simulink model "gm_am_demod_hdl_coder"  (R2021b)
settings: Solver=FixedStepAuto  StartTime=0.0  StopTime=20  RelTol=1e-3  EnableMultiTasking=on
libraries: hdlmdlgenlib x10
settings Model: Creator=caccolillo  LastModifiedBy=caccolillo
settings SolverCC: AutoInsertRateTranBlk=on
settings OptimizationCC: BlockReduction=off  ConditionallyExecuteInputs=off  DefaultParameterBehavior=Inlined  UseDivisionForNetSlopeComputation=on  GainParamInheritBuiltInType=on  UseFloatMulNetSlope=on  InlineInvariantSignals=on  EfficientFloat2IntCast=on  LifeSpan=1
settings DebuggingCC: AlgebraicLoopMsg=error  InheritedTsInSrcMsg=none  SingleTaskRateTransMsg=error
settings HardwareCC: ProdBitPerPointer=32  ProdBitPerSizeT=32  ProdBitPerPtrDiffT=32  ProdLargestAtomicFloat=None  ProdIntDivRoundTo=Undefined  ProdEndianess=Unspecified  ProdWordSize=32  ProdHWDeviceType=ASIC/FPGA->ASIC/FPGA  TargetBitPerLong=64  TargetBitPerPointer=64  TargetBitPerSizeT=64  TargetBitPerPtrDiffT=64  TargetLongLongMode=on  TargetIntDivRoundTo=Zero  TargetEndianess=LittleEndian  TargetWordSize=64  TargetHWDeviceType=Custom Processor->MATLAB Host Computer  ProdEqTarget=off
settings SFSimCC: MATLABDynamicMemAlloc=off
settings RTWCC: GenerateReport=on  LaunchReport=on
settings CodeAppCC: ForceParamTrailComments=on
settings GRTTargetCC: CombineSignalStateStructs=on  MatFileLogging=off  SupportVariableSizeSignals=on

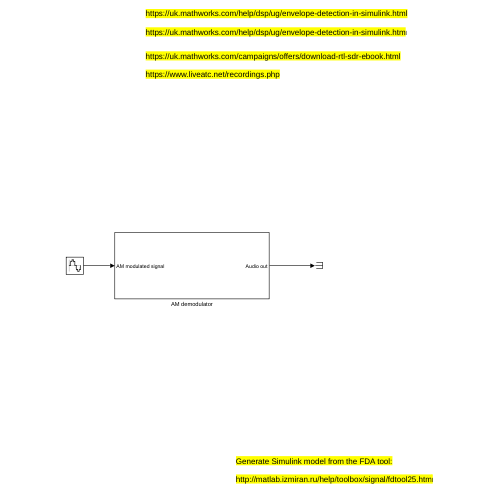
[thumbnail: Simulink's stored preview of the top-level diagram]
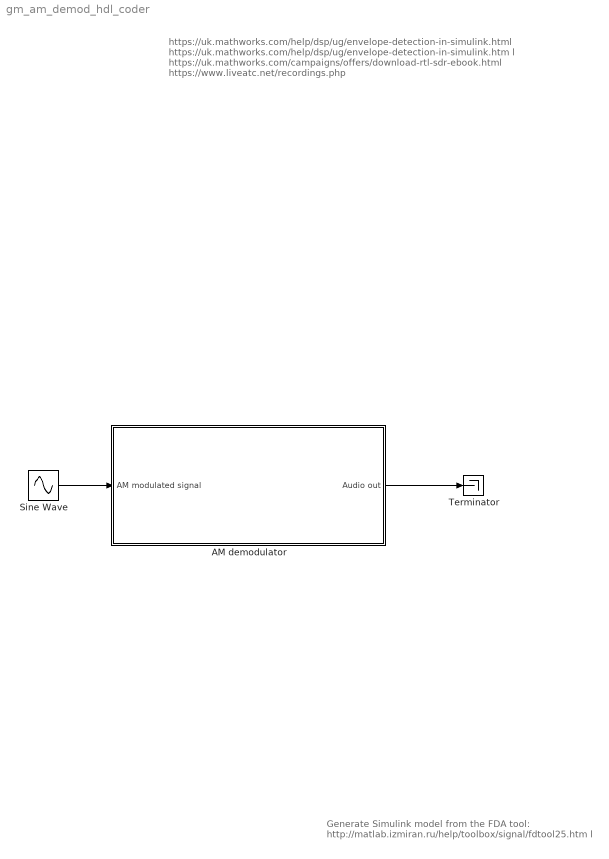
== system gm_am_demod_hdl_coder ==
  note: https://uk.mathworks.com/help/dsp/ug/envelope-detection-in-simulink.html
      |
      | https://uk.mathworks.com/help/dsp/ug/envelope-detection-in-simulink.htm l
      |
      | https://uk.mathworks.com/campaigns/offers/download-rtl-sdr-ebook.html
      |
      | https://www.liveatc.net/recordings.php
  note: Generate Simulink model from the FDA tool:
      |
      | http://matlab.izmiran.ru/help/toolbox/signal/fdtool25.htm l
  AM demodulator : Subsystem
  Sine Wave : Sin  SampleTime=1e-6
  Terminator : Terminator
  wires:
  Sine Wave/1 -> AM demodulator/1(AM modulated signal)
  AM demodulator/1(Audio out) -> Terminator/1

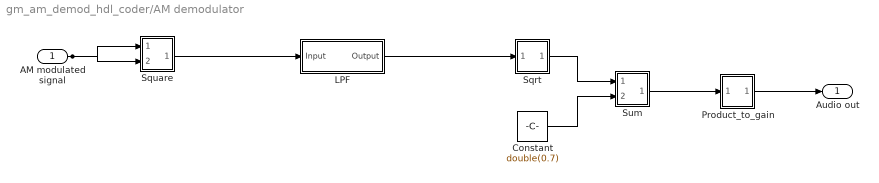
== system gm_am_demod_hdl_coder/AM demodulator ==
  AM modulated signal : Inport  OutDataTypeStr=double  PortDimensions=1  SampleTime=1e-06
  Constant : Constant  Value=double(0.7)  OutDataTypeStr=double  SampleTime=1e-06
  LPF : Subsystem
  Product_to_gain : Subsystem
      mask Display: disp('NFP\ngain_pow2');
  Sqrt : Subsystem
      mask Display: disp('NFP\nsqrt');
  Square : Subsystem
      mask Display: disp('NFP\nmul');
  Sum : Subsystem
      mask Display: disp('NFP\nadd');
  Audio out : Outport  SampleTime=1e-06
  wires:
  AM modulated signal/1 -> Square/2(In2), Square/1(In1)
  Constant/1 -> Sum/2(In2)
  LPF/1(Output) -> Sqrt/1(In1)
  Sqrt/1(Out1) -> Sum/1(In1)
  Square/1(Out1) -> LPF/1(Input)
  Sum/1(Out1) -> Product_to_gain/1(In1)
  Product_to_gain/1(Out1) -> Audio out/1

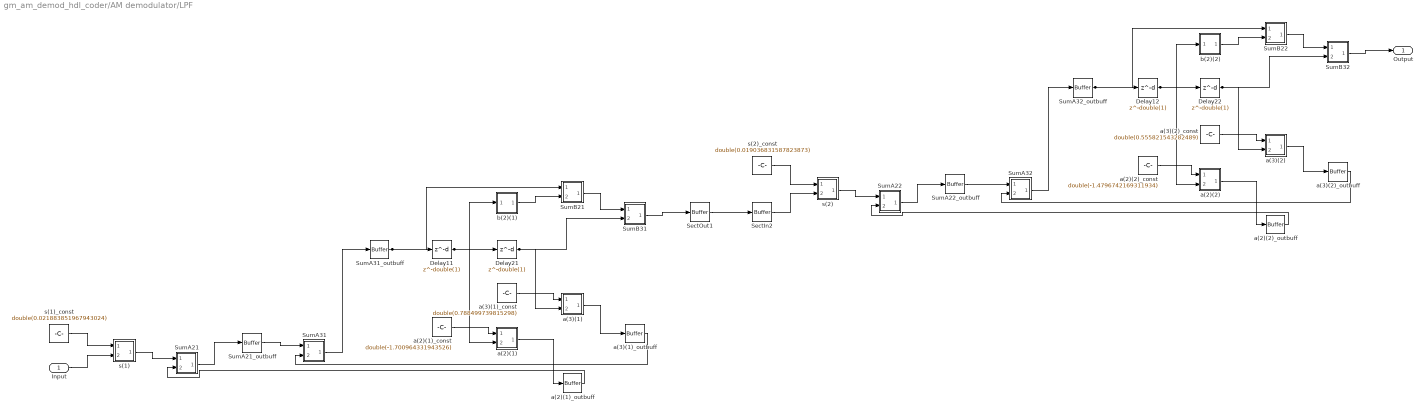
== system gm_am_demod_hdl_coder/AM demodulator/LPF ==
  Input : Inport  OutDataTypeStr=double  PortDimensions=1  SampleTime=1e-06
  Delay{11..12,21..22} (4 alike) : Delay  DelayLength=double(1)  InitialCondition=0  SampleTime=1e-06
  SectIn2 : hdlmdlgenlib/Buffer
      settings: SourceProductBaseCode=SL
  SectOut1 : hdlmdlgenlib/Buffer
      settings: SourceProductBaseCode=SL
  SumA21 : Subsystem
      mask Display: disp('NFP\nadd');
  SumA21_outbuff : hdlmdlgenlib/Buffer
      settings: SourceProductBaseCode=SL
  SumA22 : Subsystem
      mask Display: disp('NFP\nadd');
  SumA22_outbuff : hdlmdlgenlib/Buffer
      settings: SourceProductBaseCode=SL
  SumA31 : Subsystem
      mask Display: disp('NFP\nadd');
  SumA31_outbuff : hdlmdlgenlib/Buffer
      settings: SourceProductBaseCode=SL
  SumA32 : Subsystem
      mask Display: disp('NFP\nadd');
  SumA32_outbuff : hdlmdlgenlib/Buffer
      settings: SourceProductBaseCode=SL
  SumB21 : Subsystem
      mask Display: disp('NFP\nadd');
  SumB22 : Subsystem
      mask Display: disp('NFP\nadd');
  SumB31 : Subsystem
      mask Display: disp('NFP\nadd');
  SumB32 : Subsystem
      mask Display: disp('NFP\nadd');
  a(2)(1) : Subsystem
      mask Display: disp('NFP\nmul');
  a(2)(1)_const : Constant  Value=double(-1.700964331943526)  OutDataTypeStr=double  SampleTime=1e-06
  a(2)(1)_outbuff : hdlmdlgenlib/Buffer
      settings: SourceProductBaseCode=SL
  a(2)(2) : Subsystem
      mask Display: disp('NFP\nmul');
  a(2)(2)_const : Constant  Value=double(-1.4796742169311934)  OutDataTypeStr=double  SampleTime=1e-06
  a(2)(2)_outbuff : hdlmdlgenlib/Buffer
      settings: SourceProductBaseCode=SL
  a(3)(1) : Subsystem
      mask Display: disp('NFP\nmul');
  a(3)(1)_const : Constant  Value=double(0.788499739815298)  OutDataTypeStr=double  SampleTime=1e-06
  a(3)(1)_outbuff : hdlmdlgenlib/Buffer
      settings: SourceProductBaseCode=SL
  a(3)(2) : Subsystem
      mask Display: disp('NFP\nmul');
  a(3)(2)_const : Constant  Value=double(0.555821543282489)  OutDataTypeStr=double  SampleTime=1e-06
  a(3)(2)_outbuff : hdlmdlgenlib/Buffer
      settings: SourceProductBaseCode=SL
  b(2)(1) : Subsystem
      mask Display: disp('NFP\ngain_pow2');
  b(2)(2) : Subsystem
      mask Display: disp('NFP\ngain_pow2');
  s(1) : Subsystem
      mask Display: disp('NFP\nmul');
  s(1)_const : Constant  Value=double(0.021883851967943024)  OutDataTypeStr=double  SampleTime=1e-06
  s(2) : Subsystem
      mask Display: disp('NFP\nmul');
  s(2)_const : Constant  Value=double(0.019036831587823873)  OutDataTypeStr=double  SampleTime=1e-06
  Output : Outport  SampleTime=1e-06
  wires:
  Input/1 -> s(1)/2(In2)
  Delay11/1 -> a(2)(1)/2(In2), b(2)(1)/1(In1), Delay21/1
  Delay12/1 -> a(2)(2)/2(In2), b(2)(2)/1(In1), Delay22/1
  Delay21/1 -> a(3)(1)/2(In2), SumB31/2(In2)
  Delay22/1 -> a(3)(2)/2(In2), SumB32/2(In2)
  SectIn2/1 -> s(2)/2(In2)
  SumA21_outbuff/1 -> SumA31/1(In1)
  SumA22_outbuff/1 -> SumA32/1(In1)
  SumA31_outbuff/1 -> SumB21/1(In1), Delay11/1
  SumA32_outbuff/1 -> SumB22/1(In1), Delay12/1
  a(2)(1)_outbuff/1 -> SumA21/2(In2)
  a(2)(2)_outbuff/1 -> SumA22/2(In2)
  a(3)(1)_outbuff/1 -> SumA31/2(In2)
  a(3)(2)_outbuff/1 -> SumA32/2(In2)
  SectOut1/1 -> SectIn2/1
  a(2)(1)_const/1 -> a(2)(1)/1(In1)
  a(2)(2)_const/1 -> a(2)(2)/1(In1)
  a(3)(1)_const/1 -> a(3)(1)/1(In1)
  a(3)(2)_const/1 -> a(3)(2)/1(In1)
  s(1)_const/1 -> s(1)/1(In1)
  s(2)_const/1 -> s(2)/1(In1)
  b(2)(1)/1(Out1) -> SumB21/2(In2)
  b(2)(2)/1(Out1) -> SumB22/2(In2)
  SumA21/1(Out1) -> SumA21_outbuff/1
  SumA22/1(Out1) -> SumA22_outbuff/1
  SumA31/1(Out1) -> SumA31_outbuff/1
  SumA32/1(Out1) -> SumA32_outbuff/1
  SumB21/1(Out1) -> SumB31/1(In1)
  SumB22/1(Out1) -> SumB32/1(In1)
  SumB31/1(Out1) -> SectOut1/1
  SumB32/1(Out1) -> Output/1
  a(2)(1)/1(Out1) -> a(2)(1)_outbuff/1
  a(2)(2)/1(Out1) -> a(2)(2)_outbuff/1
  a(3)(1)/1(Out1) -> a(3)(1)_outbuff/1
  a(3)(2)/1(Out1) -> a(3)(2)_outbuff/1
  s(1)/1(Out1) -> SumA21/1(In1)
  s(2)/1(Out1) -> SumA22/1(In1)

== system gm_am_demod_hdl_coder/AM demodulator/Product_to_gain ==
  In1 : Inport
  Product_to_gain : Gain  Gain=double(2)
  Out1 : Outport
  wires:
  In1/1 -> Product_to_gain/1
  Product_to_gain/1 -> Out1/1

== system gm_am_demod_hdl_coder/AM demodulator/Sqrt ==
  In1 : Inport
  Sqrt : Sqrt  SampleTime=1e-06  SaturateOnIntegerOverflow=on
  Out1 : Outport
  wires:
  In1/1 -> Sqrt/1
  Sqrt/1 -> Out1/1

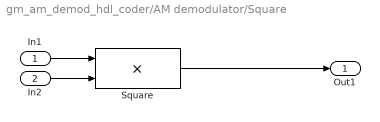
== system gm_am_demod_hdl_coder/AM demodulator/Square ==
  In1 : Inport
  In2 : Inport  Port=2
  Square : Product  Inputs=**  OutDataTypeStr=double  SampleTime=1e-06
  Out1 : Outport
  wires:
  In1/1 -> Square/1
  In2/1 -> Square/2
  Square/1 -> Out1/1

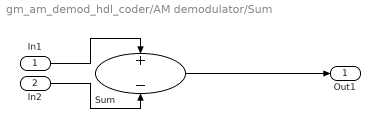
== system gm_am_demod_hdl_coder/AM demodulator/Sum ==
  In1 : Inport
  In2 : Inport  Port=2
  Sum : Sum  Inputs=+-  OutDataTypeStr=double  SampleTime=1e-06
  Out1 : Outport
  wires:
  In1/1 -> Sum/1
  In2/1 -> Sum/2
  Sum/1 -> Out1/1

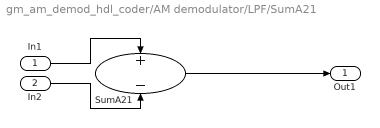
== system gm_am_demod_hdl_coder/AM demodulator/LPF/SumA21 ==
  In1 : Inport
  In2 : Inport  Port=2
  SumA21 : Sum  Inputs=+-  OutDataTypeStr=double  RndMeth=Nearest  SampleTime=1e-06
  Out1 : Outport
  wires:
  In1/1 -> SumA21/1
  In2/1 -> SumA21/2
  SumA21/1 -> Out1/1

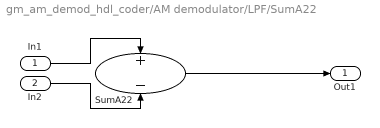
== system gm_am_demod_hdl_coder/AM demodulator/LPF/SumA22 ==
  In1 : Inport
  In2 : Inport  Port=2
  SumA22 : Sum  Inputs=+-  OutDataTypeStr=double  RndMeth=Nearest  SampleTime=1e-06
  Out1 : Outport
  wires:
  In1/1 -> SumA22/1
  In2/1 -> SumA22/2
  SumA22/1 -> Out1/1

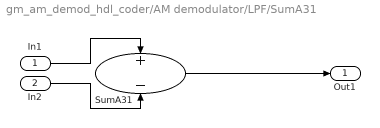
== system gm_am_demod_hdl_coder/AM demodulator/LPF/SumA31 ==
  In1 : Inport
  In2 : Inport  Port=2
  SumA31 : Sum  Inputs=+-  OutDataTypeStr=double  RndMeth=Nearest  SampleTime=1e-06
  Out1 : Outport
  wires:
  In1/1 -> SumA31/1
  In2/1 -> SumA31/2
  SumA31/1 -> Out1/1

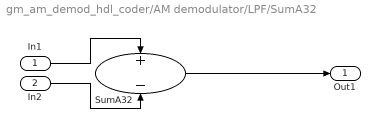
== system gm_am_demod_hdl_coder/AM demodulator/LPF/SumA32 ==
  In1 : Inport
  In2 : Inport  Port=2
  SumA32 : Sum  Inputs=+-  OutDataTypeStr=double  RndMeth=Nearest  SampleTime=1e-06
  Out1 : Outport
  wires:
  In1/1 -> SumA32/1
  In2/1 -> SumA32/2
  SumA32/1 -> Out1/1

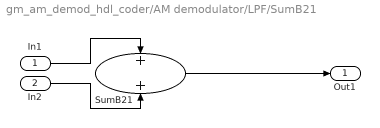
== system gm_am_demod_hdl_coder/AM demodulator/LPF/SumB21 ==
  In1 : Inport
  In2 : Inport  Port=2
  SumB21 : Sum  OutDataTypeStr=double  RndMeth=Nearest  SampleTime=1e-06
  Out1 : Outport
  wires:
  In1/1 -> SumB21/1
  In2/1 -> SumB21/2
  SumB21/1 -> Out1/1

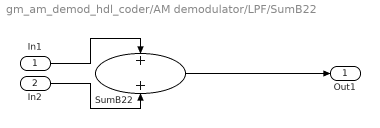
== system gm_am_demod_hdl_coder/AM demodulator/LPF/SumB22 ==
  In1 : Inport
  In2 : Inport  Port=2
  SumB22 : Sum  OutDataTypeStr=double  RndMeth=Nearest  SampleTime=1e-06
  Out1 : Outport
  wires:
  In1/1 -> SumB22/1
  In2/1 -> SumB22/2
  SumB22/1 -> Out1/1

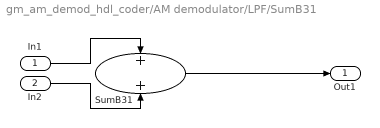
== system gm_am_demod_hdl_coder/AM demodulator/LPF/SumB31 ==
  In1 : Inport
  In2 : Inport  Port=2
  SumB31 : Sum  OutDataTypeStr=double  RndMeth=Nearest  SampleTime=1e-06
  Out1 : Outport
  wires:
  In1/1 -> SumB31/1
  In2/1 -> SumB31/2
  SumB31/1 -> Out1/1

== system gm_am_demod_hdl_coder/AM demodulator/LPF/SumB32 ==
  In1 : Inport
  In2 : Inport  Port=2
  SumB32 : Sum  OutDataTypeStr=double  RndMeth=Nearest  SampleTime=1e-06
  Out1 : Outport
  wires:
  In1/1 -> SumB32/1
  In2/1 -> SumB32/2
  SumB32/1 -> Out1/1

== system gm_am_demod_hdl_coder/AM demodulator/LPF/a(2)(1) ==
  In1 : Inport
  In2 : Inport  Port=2
  a(2)(1) : Product  Inputs=**  OutDataTypeStr=double  RndMeth=Nearest  SaturateOnIntegerOverflow=on  SampleTime=1e-06
  Out1 : Outport
  wires:
  In1/1 -> a(2)(1)/1
  In2/1 -> a(2)(1)/2
  a(2)(1)/1 -> Out1/1

== system gm_am_demod_hdl_coder/AM demodulator/LPF/a(2)(2) ==
  In1 : Inport
  In2 : Inport  Port=2
  a(2)(2) : Product  Inputs=**  OutDataTypeStr=double  RndMeth=Nearest  SaturateOnIntegerOverflow=on  SampleTime=1e-06
  Out1 : Outport
  wires:
  In1/1 -> a(2)(2)/1
  In2/1 -> a(2)(2)/2
  a(2)(2)/1 -> Out1/1

== system gm_am_demod_hdl_coder/AM demodulator/LPF/a(3)(1) ==
  In1 : Inport
  In2 : Inport  Port=2
  a(3)(1) : Product  Inputs=**  OutDataTypeStr=double  RndMeth=Nearest  SaturateOnIntegerOverflow=on  SampleTime=1e-06
  Out1 : Outport
  wires:
  In1/1 -> a(3)(1)/1
  In2/1 -> a(3)(1)/2
  a(3)(1)/1 -> Out1/1

== system gm_am_demod_hdl_coder/AM demodulator/LPF/a(3)(2) ==
  In1 : Inport
  In2 : Inport  Port=2
  a(3)(2) : Product  Inputs=**  OutDataTypeStr=double  RndMeth=Nearest  SaturateOnIntegerOverflow=on  SampleTime=1e-06
  Out1 : Outport
  wires:
  In1/1 -> a(3)(2)/1
  In2/1 -> a(3)(2)/2
  a(3)(2)/1 -> Out1/1

== system gm_am_demod_hdl_coder/AM demodulator/LPF/b(2)(1) ==
  In1 : Inport
  b(2)(1) : Gain  Gain=double(2)  RndMeth=Nearest  SaturateOnIntegerOverflow=on
  Out1 : Outport
  wires:
  In1/1 -> b(2)(1)/1
  b(2)(1)/1 -> Out1/1

== system gm_am_demod_hdl_coder/AM demodulator/LPF/b(2)(2) ==
  In1 : Inport
  b(2)(2) : Gain  Gain=double(2)  RndMeth=Nearest  SaturateOnIntegerOverflow=on
  Out1 : Outport
  wires:
  In1/1 -> b(2)(2)/1
  b(2)(2)/1 -> Out1/1

== system gm_am_demod_hdl_coder/AM demodulator/LPF/s(1) ==
  In1 : Inport
  In2 : Inport  Port=2
  s(1) : Product  Inputs=**  OutDataTypeStr=double  RndMeth=Nearest  SaturateOnIntegerOverflow=on  SampleTime=1e-06
  Out1 : Outport
  wires:
  In1/1 -> s(1)/1
  In2/1 -> s(1)/2
  s(1)/1 -> Out1/1

== system gm_am_demod_hdl_coder/AM demodulator/LPF/s(2) ==
  In1 : Inport
  In2 : Inport  Port=2
  s(2) : Product  Inputs=**  OutDataTypeStr=double  RndMeth=Nearest  SaturateOnIntegerOverflow=on  SampleTime=1e-06
  Out1 : Outport
  wires:
  In1/1 -> s(2)/1
  In2/1 -> s(2)/2
  s(2)/1 -> Out1/1
